simulink model "MPC_MG_raw_ver1"  (R2021b)
settings: Solver=ode23tb  StartTime=0.0  StopTime=1  RelTol=1e-3
model workspace (MAT data in the model file):
  Ts : Simulink.Parameter (value not decoded)
  secondary_on : Simulink.Parameter (value not decoded)
values from neighbouring files (symbols this model uses):
  A = zeros(4,4)    [MPC_MG_script_raw_dmpc.m]    (also in MPG_MG_July.m = [0 1 1 1; 1 0 0 0; 1 0 0 0; 1 0 0 0]; MPG_MG_freq_script.m = ones(4) - eye(4); Script.m = [0 1 1 1 ; 1 0 1 1 ; 1 1 0 1 ; 1 1 1 0])
  a12 = 0    [Four_DG_MG_PrimaryOnlyScript.m]    (also in MPC_MG_script_raw_dmpc.m; MPC_MG_secondary_script.m)
  a14 = 0    [Four_DG_MG_PrimaryOnlyScript.m]    (also in MPC_MG_script_raw_dmpc.m; MPC_MG_secondary_script.m)
  a21 = 1    [Four_DG_MG_PrimaryOnlyScript.m]    (also in MPC_MG_script_raw_dmpc.m; MPC_MG_secondary_script.m)
  a23 = 0    [Four_DG_MG_PrimaryOnlyScript.m]    (also in MPC_MG_script_raw_dmpc.m; MPC_MG_secondary_script.m)
  a32 = 1    [Four_DG_MG_PrimaryOnlyScript.m]    (also in MPC_MG_script_raw_dmpc.m; MPC_MG_secondary_script.m)
  a34 = 0    [Four_DG_MG_PrimaryOnlyScript.m]    (also in MPC_MG_script_raw_dmpc.m; MPC_MG_secondary_script.m)
  a41 = 1    [Four_DG_MG_PrimaryOnlyScript.m]    (also in MPC_MG_script_raw_dmpc.m; MPC_MG_secondary_script.m)
  a43 = 0    [Four_DG_MG_PrimaryOnlyScript.m]    (also in MPC_MG_script_raw_dmpc.m; MPC_MG_secondary_script.m)
  b1v = 1    [Four_DG_MG_PrimaryOnlyScript.m]    (also in MPC_MG_script_raw_dmpc.m; MPC_MG_secondary_script.m; MPG_MG_July.m; MPG_MG_freq_script.m)
  b1w = 1    [Four_DG_MG_PrimaryOnlyScript.m]    (also in MPC_MG_script_raw_dmpc.m; MPC_MG_secondary_script.m; MPG_MG_July.m; MPG_MG_freq_script.m)
  b2v = 0    [Four_DG_MG_PrimaryOnlyScript.m]    (also in MPC_MG_script_raw_dmpc.m; MPC_MG_secondary_script.m; MPG_MG_July.m; MPG_MG_freq_script.m)
  b2w = 0    [Four_DG_MG_PrimaryOnlyScript.m]    (also in MPC_MG_script_raw_dmpc.m; MPC_MG_secondary_script.m; MPG_MG_July.m; MPG_MG_freq_script.m)
  b3v = 0    [Four_DG_MG_PrimaryOnlyScript.m]    (also in MPC_MG_script_raw_dmpc.m; MPC_MG_secondary_script.m; MPG_MG_July.m; MPG_MG_freq_script.m)
  b3w = 0    [Four_DG_MG_PrimaryOnlyScript.m]    (also in MPC_MG_script_raw_dmpc.m; MPC_MG_secondary_script.m; MPG_MG_July.m; MPG_MG_freq_script.m)
  b4v = 0    [Four_DG_MG_PrimaryOnlyScript.m]    (also in MPC_MG_script_raw_dmpc.m; MPC_MG_secondary_script.m; MPG_MG_July.m; MPG_MG_freq_script.m)
  b4w = 0    [Four_DG_MG_PrimaryOnlyScript.m]    (also in MPC_MG_script_raw_dmpc.m; MPC_MG_secondary_script.m; MPG_MG_July.m; MPG_MG_freq_script.m)
  C_f = 50e-6    (= 5e-05)    [Four_DG_MG_PrimaryOnlyScript.m]    (also in MPC_MG_script.m; MPC_MG_script_raw_dmpc.m; MPC_MG_secondary_script.m; MPG_MG_July.m)
  cf = 60    [Four_DG_MG_PrimaryOnlyScript.m]    (also in MPC_MG_script_raw_dmpc.m = 40; MPC_MG_secondary_script.m = 40; MPG_MG_July.m = 100; MPG_MG_freq_script.m = 100)
  cv = 60    [Four_DG_MG_PrimaryOnlyScript.m]    (also in MPC_MG_script_raw_dmpc.m = 40; MPC_MG_secondary_script.m = 40; MPG_MG_July.m = 100; MPG_MG_freq_script.m = 100)
  f_c = 5000    [Four_DG_MG_PrimaryOnlyScript.m]    (also in MPC_MG_script.m = 40000; MPC_MG_script_raw_dmpc.m = 40000; MPC_MG_secondary_script.m = 40000; MPG_MG_July.m = 50000)
  kL = 1e-5    (= 1e-05)    [Four_DG_MG_PrimaryOnlyScript.m]    (also in MPC_MG_script.m = 1e-08; MPC_MG_script_raw_dmpc.m = 1e-08; MPC_MG_secondary_script.m = 1e-07; MPG_MG_July.m = 1e-07)
  L_f = 1.35e-3    (= 0.00135)    [Four_DG_MG_PrimaryOnlyScript.m]    (also in MPC_MG_script.m; MPC_MG_script_raw_dmpc.m; MPC_MG_secondary_script.m; MPG_MG_July.m)
  L_in1 = 0.35e-3    (= 0.00035)    [Four_DG_MG_PrimaryOnlyScript.m]    (also in MPC_MG_script.m; MPC_MG_script_raw_dmpc.m; MPC_MG_secondary_script.m; MPG_MG_July.m)
  L_in2 = 0.35e-3    (= 0.00035)    [Four_DG_MG_PrimaryOnlyScript.m]    (also in MPC_MG_script.m; MPC_MG_script_raw_dmpc.m; MPC_MG_secondary_script.m; MPG_MG_July.m)
  L_in3 = 0.35e-3    (= 0.00035)    [Four_DG_MG_PrimaryOnlyScript.m]    (also in MPC_MG_script.m; MPC_MG_script_raw_dmpc.m; MPC_MG_secondary_script.m; MPG_MG_July.m)
  lambda1 = [30000 50000 90000 50000]'    [MPC_MG_script_raw_dmpc.m]    (also in MPG_MG_July.m = [4 4 4 4]'; MPG_MG_freq_script.m = [3 3 3 3]'; Script.m = [1 1 1 1]')
  lambda2 = [5 6 7 6]'    [MPC_MG_script_raw_dmpc.m]    (also in MPG_MG_July.m = [0.5e-2 0.5e-2 0.5e-2 0.5e-2]'; MPG_MG_freq_script.m = [1.1 1.9 1.5 1.2]'; Script.m = [0.8e-2 0.8e-2 0.8e-2 0.8e-2]')
  lambda3 = [80000 80000 900000 80000]'    [MPC_MG_script_raw_dmpc.m]    (also in MPG_MG_July.m = [1e-3 1e-3 1e-3 1e-3]'; MPG_MG_freq_script.m = [9e-4 1.2e-2 3e-3 3e-3]'; Script.m = [1.5e-3 1.5e-3 1.5e-3 1.5e-3]')
  lambda4 = [5000 5000 5000 5000]'    [MPC_MG_script_raw_dmpc.m]
  lambda5 = [150 130 200 130]'    [MPC_MG_script_raw_dmpc.m]
  lambda6 = [5000 2000 1000 2000]'    [MPC_MG_script_raw_dmpc.m]
  LD_ref1 = 800e-6    (= 0.0008)    [Four_DG_MG_PrimaryOnlyScript.m]    (also in MPC_MG_script.m = 0.0003; MPC_MG_script_raw_dmpc.m = 0.0003; MPC_MG_secondary_script.m = 0.0001; MPG_MG_July.m = 0.0004)
  lo_co = 0.2    [Four_DG_MG_PrimaryOnlyScript.m]    (also in MPC_MG_script.m = 0.05; MPC_MG_script_raw_dmpc.m = 0.1; MPC_MG_secondary_script.m = 0.08; MPG_MG_July.m = 0.15)
  m_p1 = 9.4e-5/droopDivide    (= 9.4e-05)    [Four_DG_MG_PrimaryOnlyScript.m]    (also in MPC_MG_script.m; MPC_MG_script_raw_dmpc.m; MPC_MG_secondary_script.m; MPG_MG_July.m)
  m_p2 = 9.4e-5/droopDivide    (= 9.4e-05)    [Four_DG_MG_PrimaryOnlyScript.m]    (also in MPC_MG_script.m; MPC_MG_script_raw_dmpc.m; MPC_MG_secondary_script.m; MPG_MG_July.m)
  m_p3 = 12.5e-5/droopDivide    (= 0.000125)    [Four_DG_MG_PrimaryOnlyScript.m]    (also in MPC_MG_script.m; MPC_MG_script_raw_dmpc.m; MPC_MG_secondary_script.m; MPG_MG_July.m)
  m_p4 = 12.5e-5/droopDivide    (= 0.000125)    [Four_DG_MG_PrimaryOnlyScript.m]    (also in MPC_MG_script.m; MPC_MG_script_raw_dmpc.m; MPC_MG_secondary_script.m; MPG_MG_July.m)
  n_q1 = 1.3e-3/droopDivide2    (= 0.00013)    [Four_DG_MG_PrimaryOnlyScript.m]    (also in MPC_MG_script.m; MPC_MG_script_raw_dmpc.m; MPC_MG_secondary_script.m; MPG_MG_July.m)
  n_q2 = 1.3e-3/droopDivide2    (= 0.00013)    [Four_DG_MG_PrimaryOnlyScript.m]    (also in MPC_MG_script.m; MPC_MG_script_raw_dmpc.m; MPC_MG_secondary_script.m; MPG_MG_July.m)
  n_q3 = 1.5e-3/droopDivide2    (= 0.00015)    [Four_DG_MG_PrimaryOnlyScript.m]    (also in MPC_MG_script.m; MPC_MG_script_raw_dmpc.m; MPC_MG_secondary_script.m; MPG_MG_July.m)
  n_q4 = 1.5e-3/droopDivide2    (= 0.00015)    [Four_DG_MG_PrimaryOnlyScript.m]    (also in MPC_MG_script.m; MPC_MG_script_raw_dmpc.m; MPC_MG_secondary_script.m; MPG_MG_July.m)
  R_f = 0.1    [Four_DG_MG_PrimaryOnlyScript.m]    (also in MPC_MG_script.m; MPC_MG_script_raw_dmpc.m; MPC_MG_secondary_script.m; MPG_MG_July.m)
  R_in1 = 0.03    [Four_DG_MG_PrimaryOnlyScript.m]    (also in MPC_MG_script.m; MPC_MG_script_raw_dmpc.m; MPC_MG_secondary_script.m; MPG_MG_July.m)
  R_in2 = 0.03    [Four_DG_MG_PrimaryOnlyScript.m]    (also in MPC_MG_script.m; MPC_MG_script_raw_dmpc.m; MPC_MG_secondary_script.m; MPG_MG_July.m)
  R_in3 = 0.03    [Four_DG_MG_PrimaryOnlyScript.m]    (also in MPC_MG_script.m; MPC_MG_script_raw_dmpc.m; MPC_MG_secondary_script.m; MPG_MG_July.m)
  Smax = [45e3 45e3 37e3 37e3]'    [MPC_MG_script_raw_dmpc.m]
  Smax1 = 2400    [MPC_MG_script_raw_dmpc.m]
  Smax2 = 2400    [MPC_MG_script_raw_dmpc.m]
  Smax3 = 2400    [MPC_MG_script_raw_dmpc.m]
  Smax4 = 2400    [MPC_MG_script_raw_dmpc.m]
  time_thresh = 0.6    [Four_DG_MG_PrimaryOnlyScript.m]    (also in MPC_MG_script_raw_dmpc.m = 2; MPC_MG_secondary_script.m = 2; MPG_MG_July.m = 0.5; MPG_MG_freq_script.m = 0.5)
  Ts = 10e-6    (= 1e-05)    [Four_DG_MG_PrimaryOnlyScript.m]    (also in MPC_MG_script.m; MPC_MG_script_raw_dmpc.m; MPC_MG_secondary_script.m; MPG_MG_July.m)
  V_nom = 220*sqrt(2)    [Four_DG_MG_PrimaryOnlyScript.m]    (also in MPC_MG_script.m; MPC_MG_script_raw_dmpc.m; MPC_MG_secondary_script.m; MPG_MG_July.m)
  Vdc = 600    [Four_DG_MG_PrimaryOnlyScript.m]    (also in MPC_MG_script.m; MPC_MG_script_raw_dmpc.m; MPC_MG_secondary_script.m; MPG_MG_July.m)
  Vmax = 155    [MPC_MG_script_raw_dmpc.m]
  Vmin = 145    [MPC_MG_script_raw_dmpc.m]
  w_c_high = 2*pi*50    (= 314.159265359)    [Four_DG_MG_PrimaryOnlyScript.m]    (also in MPC_MG_script.m; MPC_MG_script_raw_dmpc.m; MPC_MG_secondary_script.m; MPG_MG_July.m)
  w_nom = 2*pi*50    (= 314.159265359)    [Four_DG_MG_PrimaryOnlyScript.m]    (also in MPC_MG_script.m; MPC_MG_script_raw_dmpc.m; MPC_MG_secondary_script.m; MPG_MG_July.m)
undefined symbols (not defined in the file or in its folder): i
libraries: spsThreePhaseSeriesRLCBranchLib x18, spsThreePhaseVIMeasurementLib x16, spsabctodq0Lib x16, eeGeneralControl x10, spsPLL3phLib x8, dspswit3 x5, powerlib x5, spsPMUPLLBasedPositiveSequenceLib x4, spsDCVoltageSourceLib x4, spsSeriesRLCBranchLib x4, spsTwoLevelConverterLib x4, spsThreePhaseSeriesRLCLoadLib x3
(part 4 of 4)

== matlab function MPC_MG_raw_ver1/Voltage Source Inverter 2/Model Predictive Control  ==
  settings: updateMethod=DISCRETE  sampleTime=Ts
  data: S_opt output; Sopt output size=[1 6]; Vc input; i_filter input; vref input; Vi_opt output; Vdc parameter double size=1; modT parameter size=1; Cfilter parameter size=1; Lfilter parameter size=1
function [S_opt, Sopt, Vi_opt] = MPC(Vc, i_filter,vref,Vdc,modT,Cfilter,Lfilter)

    % In order to call "cont2dis" function
    coder.extrinsic('cont2dis');
    persistent Aq Bq Bdq Vck ifk  Vc_old if_old x_opt g f_window f_window2

    % Initialize variables and get the parameters of the Discrete model based on Ts
    if isempty(x_opt), x_opt = ones(1, 2); end
    if isempty(Vc_old), Vc_old = 0 + 1j*0; end
    if isempty(if_old), if_old = 0 + 1j*0; end
    if isempty(Vck), Vck = ones(1, 4) * (0 + 1j*0); end
    if isempty(ifk), ifk = ones(1, 4) * (0 + 1j*0); end
    if isempty(f_window), f_window = zeros(1,51); end
    if isempty(f_window2), f_window2 = zeros(1,51); end

    if isempty(Aq) && isempty(Bq) && isempty(Bdq)
        Aq = zeros(2);     Bq = zeros(2,1);     Bdq = zeros(2,1);
        % Call "cont2dis" function
        [Aq, Bq, Bdq] = cont2dis(modT,Lfilter,Cfilter); 
    end
    
    % Intialize the cost function
    g_opt = inf;
    
    % To generate the switching states matrix
    states = [1 0 0;
              0 0 0  
              1 1 0
              0 1 0
              0 1 1
              0 0 1
              1 0 1
              1 1 1];
    a = exp(1j*(2*pi/3));
    % Read current measurements at sampling instant k
    ifk(1) = i_filter;
    Vck(1) = Vc;
    % Equation of io(k-1) = if(k-1)-(c/Ts)(vc(k)-vc(k-1)).
    io = ones(1, 3) * (0 + 1j*0);
    io(1) = if_old - (Cfilter/modT)*(Vck(1) - Vc_old); 
    
    % Store the measured current for the next iteration
    if_old = i_filter;
    Vc_old = Vc;
    % FOR loop to find the best switch in the next instant and its corresponding V(i)
    k = ones(1,3);
    s = zeros(3,3);
    sw = zeros(1,3)* (0 + 1j*0);
    Vi = zeros(1,3)* (0 + 1j*0);
    for a1 = 1:8
        k(1) = a1;
        %constraint check
        if (abs(states(k(1),:)-states(x_opt(1),:)) > 1)
            continue
        end
        %state calculation
        s(1,:) = states(k(1),:);
        sw(1) = (2/3)*(s(1,1)+a*s(1,2)+a^2*s(1,3));
        Vi(1) = Vdc*sw(1);

        % Output Voltage Prediction at instant k+1
        ifk(2) = Aq(1,1)*ifk(1) + Aq(1,2)*Vck(1) + Bq(1)*Vi(1) + Bdq(1)*io(1); 
        Vck(2) = Aq(2,1)*ifk(1) + Aq(2,2)*Vck(1) + Bq(2)*Vi(1) + Bdq(2)*io(1); 
        
        for a2 = 1:8
            k(2) = a2;
            %constraint check
            if (abs(states(k(2),:)-states(k(1),:)) > 1)
                continue
            end
            io(2) = io(1) - (Cfilter/modT)*(Vck(2) - Vck(1));
            %state calculation
            s(2,:) = states(k(2),:);
            sw(2) = (2/3)*(s(2,1)+a*s(2,2)+a^2*s(2,3));
            Vi(2) = Vdc*sw(2);
    
            % Output Voltage Prediction at instant k+1
            ifk(3) = Aq(1,1)*ifk(2) + Aq(1,2)*Vck(2) + Bq(1)*Vi(2) + Bdq(1)*io(2); 
            Vck(3) = Aq(2,1)*ifk(2) + Aq(2,2)*Vck(2) + Bq(2)*Vi(2) + Bdq(2)*io(2); 

            g1 = (real(ifk(3))-real(io(3))+Cfilter*2*pi*50*imag(vref))^2 + (imag(ifk(3))-imag(io(3))+Cfilter*2*pi*50*real(vref))^2;
            g = (real(vref)-real(Vck(3)))^2+(imag(vref)-imag(Vck(3)))^2 + 0.1*g1;
            if (g<g_opt)
                x_opt = [k(1) k(2)];
                g_opt = g;
            end
           
        end 
    end

     
    
    % Output switching states and its voltage vector. 
    Vi_opt = x_opt(1); 
    S_opt = states(x_opt(1),:);
    d_opt = not(S_opt);
    Sopt = [S_opt,d_opt];     

end

== matlab function MPC_MG_raw_ver1/Voltage Source Inverter 1/Model Predictive Control  ==
  settings: updateMethod=DISCRETE  sampleTime=Ts
  data: S_opt output; Sopt output size=[1 6]; Vc input; i_filter input; vref input; Vi_opt output; Vdc parameter double size=1; modT parameter size=1; Cfilter parameter size=1; Lfilter parameter size=1
function [S_opt, Sopt, Vi_opt] = MPC(Vc, i_filter,vref,Vdc,modT,Cfilter,Lfilter)

    % In order to call "cont2dis" function
    coder.extrinsic('cont2dis');
    persistent Aq Bq Bdq Vck ifk  Vc_old if_old x_opt g f_window f_window2

    % Initialize variables and get the parameters of the Discrete model based on Ts
    if isempty(x_opt), x_opt = ones(1, 2); end
    if isempty(Vc_old), Vc_old = 0 + 1j*0; end
    if isempty(if_old), if_old = 0 + 1j*0; end
    if isempty(Vck), Vck = ones(1, 4) * (0 + 1j*0); end
    if isempty(ifk), ifk = ones(1, 4) * (0 + 1j*0); end
    if isempty(f_window), f_window = zeros(1,51); end
    if isempty(f_window2), f_window2 = zeros(1,51); end

    if isempty(Aq) && isempty(Bq) && isempty(Bdq)
        Aq = zeros(2);     Bq = zeros(2,1);     Bdq = zeros(2,1);
        % Call "cont2dis" function
        [Aq, Bq, Bdq] = cont2dis(modT,Lfilter,Cfilter); 
    end
    
    % Intialize the cost function
    g_opt = inf;
    
    % To generate the switching states matrix
    states = [1 0 0;
              0 0 0  
              1 1 0
              0 1 0
              0 1 1
              0 0 1
              1 0 1
              1 1 1];
    a = exp(1j*(2*pi/3));
    % Read current measurements at sampling instant k
    ifk(1) = i_filter;
    Vck(1) = Vc;
    % Equation of io(k-1) = if(k-1)-(c/Ts)(vc(k)-vc(k-1)).
    io = ones(1, 3) * (0 + 1j*0);
    io(1) = if_old - (Cfilter/modT)*(Vck(1) - Vc_old); 
    
    % Store the measured current for the next iteration
    if_old = i_filter;
    Vc_old = Vc;
    % FOR loop to find the best switch in the next instant and its corresponding V(i)
    k = ones(1,3);
    s = zeros(3,3);
    sw = zeros(1,3)* (0 + 1j*0);
    Vi = zeros(1,3)* (0 + 1j*0);
    for a1 = 1:8
        k(1) = a1;
        %constraint check
        if (abs(states(k(1),:)-states(x_opt(1),:)) > 1)
            continue
        end
        %state calculation
        s(1,:) = states(k(1),:);
        sw(1) = (2/3)*(s(1,1)+a*s(1,2)+a^2*s(1,3));
        Vi(1) = Vdc*sw(1);

        % Output Voltage Prediction at instant k+1
        ifk(2) = Aq(1,1)*ifk(1) + Aq(1,2)*Vck(1) + Bq(1)*Vi(1) + Bdq(1)*io(1); 
        Vck(2) = Aq(2,1)*ifk(1) + Aq(2,2)*Vck(1) + Bq(2)*Vi(1) + Bdq(2)*io(1); 
        
        for a2 = 1:8
            k(2) = a2;
            %constraint check
            if (abs(states(k(2),:)-states(k(1),:)) > 1)
                continue
            end
            io(2) = io(1) - (Cfilter/modT)*(Vck(2) - Vck(1));
            %state calculation
            s(2,:) = states(k(2),:);
            sw(2) = (2/3)*(s(2,1)+a*s(2,2)+a^2*s(2,3));
            Vi(2) = Vdc*sw(2);
    
            % Output Voltage Prediction at instant k+1
            ifk(3) = Aq(1,1)*ifk(2) + Aq(1,2)*Vck(2) + Bq(1)*Vi(2) + Bdq(1)*io(2); 
            Vck(3) = Aq(2,1)*ifk(2) + Aq(2,2)*Vck(2) + Bq(2)*Vi(2) + Bdq(2)*io(2); 

            g1 = (real(ifk(3))-real(io(3))+Cfilter*2*pi*50*imag(vref))^2 + (imag(ifk(3))-imag(io(3))+Cfilter*2*pi*50*real(vref))^2;
            g = (real(vref)-real(Vck(3)))^2+(imag(vref)-imag(Vck(3)))^2 + 0.1*g1;
            if (g<g_opt)
                x_opt = [k(1) k(2)];
                g_opt = g;
            end
           
        end 
    end

     
    
    % Output switching states and its voltage vector. 
    Vi_opt = x_opt(1); 
    S_opt = states(x_opt(1),:);
    d_opt = not(S_opt);
    Sopt = [S_opt,d_opt];     

end

== matlab function MPC_MG_raw_ver1/Voltage Source Inverter 3/Model Predictive Control  ==
  settings: updateMethod=DISCRETE  sampleTime=Ts
  data: S_opt output; Sopt output size=[1 6]; Vc input; i_filter input; vref input; Vi_opt output; Vdc parameter double size=1; modT parameter size=1; Cfilter parameter size=1; Lfilter parameter size=1
function [S_opt, Sopt, Vi_opt] = MPC(Vc, i_filter,vref,Vdc,modT,Cfilter,Lfilter)

    % In order to call "cont2dis" function
    coder.extrinsic('cont2dis');
    persistent Aq Bq Bdq Vck ifk  Vc_old if_old x_opt g f_window f_window2

    % Initialize variables and get the parameters of the Discrete model based on Ts
    if isempty(x_opt), x_opt = ones(1, 2); end
    if isempty(Vc_old), Vc_old = 0 + 1j*0; end
    if isempty(if_old), if_old = 0 + 1j*0; end
    if isempty(Vck), Vck = ones(1, 4) * (0 + 1j*0); end
    if isempty(ifk), ifk = ones(1, 4) * (0 + 1j*0); end
    if isempty(f_window), f_window = zeros(1,51); end
    if isempty(f_window2), f_window2 = zeros(1,51); end

    if isempty(Aq) && isempty(Bq) && isempty(Bdq)
        Aq = zeros(2);     Bq = zeros(2,1);     Bdq = zeros(2,1);
        % Call "cont2dis" function
        [Aq, Bq, Bdq] = cont2dis(modT,Lfilter,Cfilter); 
    end
    
    % Intialize the cost function
    g_opt = inf;
    
    % To generate the switching states matrix
    states = [1 0 0;
              0 0 0  
              1 1 0
              0 1 0
              0 1 1
              0 0 1
              1 0 1
              1 1 1];
    a = exp(1j*(2*pi/3));
    % Read current measurements at sampling instant k
    ifk(1) = i_filter;
    Vck(1) = Vc;
    % Equation of io(k-1) = if(k-1)-(c/Ts)(vc(k)-vc(k-1)).
    io = ones(1, 3) * (0 + 1j*0);
    io(1) = if_old - (Cfilter/modT)*(Vck(1) - Vc_old); 
    
    % Store the measured current for the next iteration
    if_old = i_filter;
    Vc_old = Vc;
    % FOR loop to find the best switch in the next instant and its corresponding V(i)
    k = ones(1,3);
    s = zeros(3,3);
    sw = zeros(1,3)* (0 + 1j*0);
    Vi = zeros(1,3)* (0 + 1j*0);
    for a1 = 1:8
        k(1) = a1;
        %constraint check
        if (abs(states(k(1),:)-states(x_opt(1),:)) > 1)
            continue
        end
        %state calculation
        s(1,:) = states(k(1),:);
        sw(1) = (2/3)*(s(1,1)+a*s(1,2)+a^2*s(1,3));
        Vi(1) = Vdc*sw(1);

        % Output Voltage Prediction at instant k+1
        ifk(2) = Aq(1,1)*ifk(1) + Aq(1,2)*Vck(1) + Bq(1)*Vi(1) + Bdq(1)*io(1); 
        Vck(2) = Aq(2,1)*ifk(1) + Aq(2,2)*Vck(1) + Bq(2)*Vi(1) + Bdq(2)*io(1); 
        
        for a2 = 1:8
            k(2) = a2;
            %constraint check
            if (abs(states(k(2),:)-states(k(1),:)) > 1)
                continue
            end
            io(2) = io(1) - (Cfilter/modT)*(Vck(2) - Vck(1));
            %state calculation
            s(2,:) = states(k(2),:);
            sw(2) = (2/3)*(s(2,1)+a*s(2,2)+a^2*s(2,3));
            Vi(2) = Vdc*sw(2);
    
            % Output Voltage Prediction at instant k+1
            ifk(3) = Aq(1,1)*ifk(2) + Aq(1,2)*Vck(2) + Bq(1)*Vi(2) + Bdq(1)*io(2); 
            Vck(3) = Aq(2,1)*ifk(2) + Aq(2,2)*Vck(2) + Bq(2)*Vi(2) + Bdq(2)*io(2); 

            g1 = (real(ifk(3))-real(io(3))+Cfilter*2*pi*50*imag(vref))^2 + (imag(ifk(3))-imag(io(3))+Cfilter*2*pi*50*real(vref))^2;
            g = (real(vref)-real(Vck(3)))^2+(imag(vref)-imag(Vck(3)))^2 + 0.1*g1;
            if (g<g_opt)
                x_opt = [k(1) k(2)];
                g_opt = g;
            end
           
        end 
    end

     
    
    % Output switching states and its voltage vector. 
    Vi_opt = x_opt(1); 
    S_opt = states(x_opt(1),:);
    d_opt = not(S_opt);
    Sopt = [S_opt,d_opt];     

end

== matlab function MPC_MG_raw_ver1/MPC-based Secondary Controller/Model Predictive Control 1 ==
  settings: updateMethod=DISCRETE  sampleTime=Ts
  data: L_f input; Mpw input; Mqv input; Tsec input; omega input; omega_s input; V input; V_s input; theta input; d_omega output; d_V output size=[1 6]; P input; Q input; a input; Vmin input; Vmax input; w_nom input; V_nom input; lambda1 input; lambda2 input; lambda3 input; lambda4 input; lambda5 input; lambda6 input; Smax input; aij input
function [d_omega, d_V] = fcn(L_f, Mpw, Mqv, Tsec, omega, omega_s, V, V_s, theta, P, Q, a, Vmin, Vmax, w_nom, V_nom, lambda1, lambda2, lambda3, lambda4, lambda5, lambda6, Smax, aij)
    persistent omega_k V_k theta_k P_k Q_k d_omega_old d_V_old;
    
    if isempty(omega_k), omega_k = 0; end
    if isempty(V_k), V_k = 0; end
    if isempty(theta_k), theta_k = 0; end
    if isempty(P_k), P_k = 0; end
    if isempty(Q_k), Q_k = 0; end
    if isempty(d_omega_old), d_omega_old = 0; end
    if isempty(d_V_old), d_V_old = 0; end
    %all inputs are 4-element vector
    %step 4:
    %omega_overline = (omega(a) + aij(a,:)*omega)/ (1+aij(a,:));
    %V_overline = (V(a) + aij(a,:)*V)/ (1+aij(a,:));
    %step 5: update matrices
    Ai = zeros(3,9);
    Ai(1,4) = 1;
    Ai(2,4) = -1;
    Ai(3,5) = sign(P(a));
    Ai(3,6) = sign(Q(a));
    
    Bi = zeros(3,1);
    Bi(1,1) = Vmin;
    Bi(2,1) = -Vmax;
    Bi(3,1) = Smax(a) -(abs(P(a))+abs(Q(a))) + sign(P(a))*P(a) + sign(Q(a))*Q(a);

    omega_k = omega(a) + Mpw*(P_k - P(a)) + d_omega_old;
    V_k = V(a) + Mqv*(Q_k - Q(a)) + d_V_old;
    theta_k = theta + Tsec*(omega_k - omega_s(a));
    P_k = P(a) + (V_k - V(a))/(L_f*w_nom)*V_s(a)*sin(theta(a)) + (theta_k-theta(a))/(L_f*w_nom)*V(a)*V_s(a)*cos(theta(a));
    Q_k = Q(a) + (V_k - V(a))/(L_f*w_nom)*(2*V(a)-V_s(a)*cos(theta(a))) + (theta_k-theta(a))/(L_f*w_nom)*V(a)*V_s(a)*sin(theta(a));
    Aeq = eye(7,9);
    Beq = [w_nom; V_nom; omega_k; V_k; theta_k; P_k; Q_k ; 0; 0];
    
    H = zeros(9);
    H(1,1) = 2*lambda1(a);
    H(2,2) = 2*lambda2(a);
    H(6,6) = 2*lambda5(a)/Smax(a);
    H(7,7) = H(6,6)*lambda6(a)/lambda5(a);
    H(8,8) = 2*lambda3(a);
    H(9,9) = 2*lambda4(a);
    
    F = zeros(9,1);
    F(1,1) = -2*lambda1(a);
    F(2,1) = -2*lambda2(a);
    F(6,1) = -2*lambda5(a)*sum(aij(a,:)*P/Smax)*P(a)/Smax(a);
    F(7,1) = -2*lambda6(a)*sum(aij(a,:)*P/Smax)*P(a)/Smax(a);

    options = optimoptions('quadprog','Display','iter');

    [x, exitflag] = quadprog(H, F, Ai, Bi, Aeq, Beq, [], [], [], options);

    if exitflag > 0
        d_omega = x(8);
        d_V = x(9);
    else
        d_omega = 0;
        d_V = 0;
    end
    d_omega_old = d_omega;
    d_V_old = d_V;
    
end

== matlab function MPC_MG_raw_ver1/Voltage Source Inverter 5/Model Predictive Control  ==
  settings: updateMethod=DISCRETE  sampleTime=Ts
  data: S_opt output; Sopt output size=[1 6]; Vc input; i_filter input; vref input; Vi_opt output; Vdc parameter double size=1; modT parameter size=1; Cfilter parameter size=1; Lfilter parameter size=1
function [S_opt, Sopt, Vi_opt] = MPC(Vc, i_filter,vref,Vdc,modT,Cfilter,Lfilter)

    % In order to call "cont2dis" function
    coder.extrinsic('cont2dis');
    persistent Aq Bq Bdq Vc1 if1 Vc_old if_old x_opt g f_window f_window2 fil fil2

    % Initialize variables and get the parameters of the Discrete model based on Ts
    if isempty(x_opt), x_opt = 1; end
    if isempty(Vc1), Vc1 = 0 + 1j*0; end
    if isempty(Vc_old), Vc_old = 0 + 1j*0; end
    if isempty(if_old), if_old = 0 + 1j*0; end
    if isempty(if1), if1 = 0 + 1j*0; end
    if isempty(f_window), f_window = zeros(1,51); end
    if isempty(f_window2), f_window2 = zeros(1,51); end

    if isempty(Aq) && isempty(Bq) && isempty(Bdq)
        Aq = zeros(2);     Bq = zeros(2,1);     Bdq = zeros(2,1);
        % Call "cont2dis" function
        [Aq, Bq, Bdq] = cont2dis(modT,Lfilter,Cfilter); 
    end
    
    % Intialize the cost function
    g_opt = inf;
    
    % To generate the switching states matrix
    states = [1 0 0;
              0 0 0  
              1 1 0
              0 1 0
              0 1 1
              0 0 1
              1 0 1
              1 1 1];
    a = exp(1j*(2*pi/3));
    %notch filter
    fil = fir1(2,[0.1225 0.1275],'DC-0');
    fil2 = fir1(2,[0.1225 0.1275],'DC-0');
    
    % Read current measurements at sampling instant k
    ifk = i_filter;
    Vck = Vc;
    % Equation of io(k-1) = if(k-1)-(c/Ts)(vc(k)-vc(k-1)).
    io = if_old - (Cfilter/modT)*(Vck - Vc_old); 
    
    % Store the measured current for the next iteration
    if_old = ifk;
    Vc_old = Vck;
    % FOR loop to find the best switch in the next instant and its corresponding V(i)
    for k = 1:8
        s = states(k,:);
        sw = (2/3)*(s(1)+a*s(2)+a^2*s(3));
        Vi = Vdc*sw;

        % Output Voltage Prediction at instant k+1
        if1 = Aq(1,1)*ifk + Aq(1,2)*Vck + Bq(1)*Vi + Bdq(1)*io; 
        Vc1 = Aq(2,1)*ifk + Aq(2,2)*Vck + Bq(2)*Vi + Bdq(2)*io; 
        Nc = sum(abs(states(k,:)-states(x_opt,:)))^2;    
        gf = filter(fil, 1, f_window);
        gf2 = filter(fil2, 1, f_window2);
        g1 = (real(if1)-real(io)+Cfilter*2*pi*50*imag(vref))^2 + (imag(if1)-imag(io)+Cfilter*2*pi*50*real(vref))^2;
        g = (real(vref)-real(Vc1))^2+(imag(vref)-imag(Vc1))^2 + 0.1*g1 + 3*Nc + 3*gf(1) + 3*gf2(1);
        if (g < g_opt)
            x_opt = k;
            g_opt = g;
            f_window = [sqrt((real(vref)-real(Vc1))^2+(imag(vref)-imag(Vc1))^2), f_window(1:(length(f_window)-1))];
            f_window2 = [g, f_window2(1:(length(f_window2)-1))];
        end
             
    end
    
    % Output switching states and its voltage vector. 
    Vi_opt = x_opt; 
    S_opt = states(x_opt,:);
    d_opt = not(S_opt);
    Sopt = [S_opt,d_opt];     

end

== matlab function MPC_MG_raw_ver1/MPC-based Secondary Controller/Model Predictive Control 2 ==
  settings: updateMethod=DISCRETE  sampleTime=Ts
  data: L_f input; Mpw input; Mqv input; Tsec input; omega input; omega_s input; V input; V_s input; theta input; d_omega output; d_V output size=[1 6]; P input; Q input; a input; Vmin input; Vmax input; w_nom input; V_nom input; lambda1 input; lambda2 input; lambda3 input; lambda4 input; lambda5 input; lambda6 input; Smax input; aij input
function [d_omega, d_V] = fcn(L_f, Mpw, Mqv, Tsec, omega, omega_s, V, V_s, theta, P, Q, a, Vmin, Vmax, w_nom, V_nom, lambda1, lambda2, lambda3, lambda4, lambda5, lambda6, Smax, aij)
    persistent omega_k V_k theta_k P_k Q_k d_omega_old d_V_old;
    
    if isempty(omega_k), omega_k = 0; end
    if isempty(V_k), V_k = 0; end
    if isempty(theta_k), theta_k = 0; end
    if isempty(P_k), P_k = 0; end
    if isempty(Q_k), Q_k = 0; end
    if isempty(d_omega_old), d_omega_old = 0; end
    if isempty(d_V_old), d_V_old = 0; end
    %all inputs are 4-element vector
    %step 4:
    %omega_overline = (omega(a) + aij(a,:)*omega)/ (1+aij(a,:));
    %V_overline = (V(a) + aij(a,:)*V)/ (1+aij(a,:));
    %step 5: update matrices
    Ai = zeros(3,9);
    Ai(1,4) = 1;
    Ai(2,4) = -1;
    Ai(3,5) = sign(P(a));
    Ai(3,6) = sign(Q(a));
    
    Bi = zeros(3,1);
    Bi(1,1) = Vmin;
    Bi(2,1) = -Vmax;
    Bi(3,1) = Smax(a) -(abs(P(a))+abs(Q(a))) + sign(P(a))*P(a) + sign(Q(a))*Q(a);

    omega_k = omega(a) + Mpw*(P_k - P(a)) + d_omega_old;
    V_k = V(a) + Mqv*(Q_k - Q(a)) + d_V_old;
    theta_k = theta + Tsec*(omega_k - omega_s(a));
    P_k = P(a) + (V_k - V(a))/(L_f*w_nom)*V_s(a)*sin(theta(a)) + (theta_k-theta(a))/(L_f*w_nom)*V(a)*V_s(a)*cos(theta(a));
    Q_k = Q(a) + (V_k - V(a))/(L_f*w_nom)*(2*V(a)-V_s(a)*cos(theta(a))) + (theta_k-theta(a))/(L_f*w_nom)*V(a)*V_s(a)*sin(theta(a));
    Aeq = eye(7,9);
    Beq = [w_nom; V_nom; omega_k; V_k; theta_k; P_k; Q_k ; 0; 0];
    
    H = zeros(9);
    H(1,1) = 2*lambda1(a);
    H(2,2) = 2*lambda2(a);
    H(6,6) = 2*lambda5(a)/Smax(a);
    H(7,7) = H(6,6)*lambda6(a)/lambda5(a);
    H(8,8) = 2*lambda3(a);
    H(9,9) = 2*lambda4(a);
    
    F = zeros(9,1);
    F(1,1) = -2*lambda1(a);
    F(2,1) = -2*lambda2(a);
    F(6,1) = -2*lambda5(a)*sum(aij(a,:)*P/Smax)*P(a)/Smax(a);
    F(7,1) = -2*lambda6(a)*sum(aij(a,:)*P/Smax)*P(a)/Smax(a);

    options = optimoptions('quadprog','Display','iter');

    [x, exitflag] = quadprog(H, F, Ai, Bi, Aeq, Beq, [], [], [], options);

    if exitflag > 0
        d_omega = x(8);
        d_V = x(9);
    else
        d_omega = 0;
        d_V = 0;
    end
    d_omega_old = d_omega;
    d_V_old = d_V;
    
end

== matlab function MPC_MG_raw_ver1/MPC-based Secondary Controller/Model Predictive Control 3 ==
  settings: updateMethod=DISCRETE  sampleTime=Ts
  data: L_f input; Mpw input; Mqv input; Tsec input; omega input; omega_s input; V input; V_s input; theta input; d_omega output; d_V output size=[1 6]; P input; Q input; a input; Vmin input; Vmax input; w_nom input; V_nom input; lambda1 input; lambda2 input; lambda3 input; lambda4 input; lambda5 input; lambda6 input; Smax input; aij input
function [d_omega, d_V] = fcn(L_f, Mpw, Mqv, Tsec, omega, omega_s, V, V_s, theta, P, Q, a, Vmin, Vmax, w_nom, V_nom, lambda1, lambda2, lambda3, lambda4, lambda5, lambda6, Smax, aij)
    persistent omega_k V_k theta_k P_k Q_k d_omega_old d_V_old;
    
    if isempty(omega_k), omega_k = 0; end
    if isempty(V_k), V_k = 0; end
    if isempty(theta_k), theta_k = 0; end
    if isempty(P_k), P_k = 0; end
    if isempty(Q_k), Q_k = 0; end
    if isempty(d_omega_old), d_omega_old = 0; end
    if isempty(d_V_old), d_V_old = 0; end
    %all inputs are 4-element vector
    %step 4:
    %omega_overline = (omega(a) + aij(a,:)*omega)/ (1+aij(a,:));
    %V_overline = (V(a) + aij(a,:)*V)/ (1+aij(a,:));
    %step 5: update matrices
    Ai = zeros(3,9);
    Ai(1,4) = 1;
    Ai(2,4) = -1;
    Ai(3,5) = sign(P(a));
    Ai(3,6) = sign(Q(a));
    
    Bi = zeros(3,1);
    Bi(1,1) = Vmin;
    Bi(2,1) = -Vmax;
    Bi(3,1) = Smax(a) -(abs(P(a))+abs(Q(a))) + sign(P(a))*P(a) + sign(Q(a))*Q(a);

    omega_k = omega(a) + Mpw*(P_k - P(a)) + d_omega_old;
    V_k = V(a) + Mqv*(Q_k - Q(a)) + d_V_old;
    theta_k = theta + Tsec*(omega_k - omega_s(a));
    P_k = P(a) + (V_k - V(a))/(L_f*w_nom)*V_s(a)*sin(theta(a)) + (theta_k-theta(a))/(L_f*w_nom)*V(a)*V_s(a)*cos(theta(a));
    Q_k = Q(a) + (V_k - V(a))/(L_f*w_nom)*(2*V(a)-V_s(a)*cos(theta(a))) + (theta_k-theta(a))/(L_f*w_nom)*V(a)*V_s(a)*sin(theta(a));
    Aeq = eye(7,9);
    Beq = [w_nom; V_nom; omega_k; V_k; theta_k; P_k; Q_k ; 0; 0];
    
    H = zeros(9);
    H(1,1) = 2*lambda1(a);
    H(2,2) = 2*lambda2(a);
    H(6,6) = 2*lambda5(a)/Smax(a);
    H(7,7) = H(6,6)*lambda6(a)/lambda5(a);
    H(8,8) = 2*lambda3(a);
    H(9,9) = 2*lambda4(a);
    
    F = zeros(9,1);
    F(1,1) = -2*lambda1(a);
    F(2,1) = -2*lambda2(a);
    F(6,1) = -2*lambda5(a)*sum(aij(a,:)*P/Smax)*P(a)/Smax(a);
    F(7,1) = -2*lambda6(a)*sum(aij(a,:)*P/Smax)*P(a)/Smax(a);

    options = optimoptions('quadprog','Display','iter');

    [x, exitflag] = quadprog(H, F, Ai, Bi, Aeq, Beq, [], [], [], options);

    if exitflag > 0
        d_omega = x(8);
        d_V = x(9);
    else
        d_omega = 0;
        d_V = 0;
    end
    d_omega_old = d_omega;
    d_V_old = d_V;
    
end

== matlab function MPC_MG_raw_ver1/Voltage Source Inverter 4/Model Predictive Control  ==
  settings: updateMethod=DISCRETE  sampleTime=Ts
  data: S_opt output; Sopt output size=[1 6]; Vc input; i_filter input; vref input; Vi_opt output; Vdc parameter double size=1; modT parameter size=1; Cfilter parameter size=1; Lfilter parameter size=1
function [S_opt, Sopt, Vi_opt] = MPC(Vc, i_filter,vref,Vdc,modT,Cfilter,Lfilter)

    % In order to call "cont2dis" function
    coder.extrinsic('cont2dis');
    persistent Aq Bq Bdq Vck ifk  Vc_old if_old x_opt g f_window f_window2

    % Initialize variables and get the parameters of the Discrete model based on Ts
    if isempty(x_opt), x_opt = ones(1, 2); end
    if isempty(Vc_old), Vc_old = 0 + 1j*0; end
    if isempty(if_old), if_old = 0 + 1j*0; end
    if isempty(Vck), Vck = ones(1, 4) * (0 + 1j*0); end
    if isempty(ifk), ifk = ones(1, 4) * (0 + 1j*0); end
    if isempty(f_window), f_window = zeros(1,51); end
    if isempty(f_window2), f_window2 = zeros(1,51); end

    if isempty(Aq) && isempty(Bq) && isempty(Bdq)
        Aq = zeros(2);     Bq = zeros(2,1);     Bdq = zeros(2,1);
        % Call "cont2dis" function
        [Aq, Bq, Bdq] = cont2dis(modT,Lfilter,Cfilter); 
    end
    
    % Intialize the cost function
    g_opt = inf;
    
    % To generate the switching states matrix
    states = [1 0 0;
              0 0 0  
              1 1 0
              0 1 0
              0 1 1
              0 0 1
              1 0 1
              1 1 1];
    a = exp(1j*(2*pi/3));
    % Read current measurements at sampling instant k
    ifk(1) = i_filter;
    Vck(1) = Vc;
    % Equation of io(k-1) = if(k-1)-(c/Ts)(vc(k)-vc(k-1)).
    io = ones(1, 3) * (0 + 1j*0);
    io(1) = if_old - (Cfilter/modT)*(Vck(1) - Vc_old); 
    
    % Store the measured current for the next iteration
    if_old = i_filter;
    Vc_old = Vc;
    % FOR loop to find the best switch in the next instant and its corresponding V(i)
    k = ones(1,3);
    s = zeros(3,3);
    sw = zeros(1,3)* (0 + 1j*0);
    Vi = zeros(1,3)* (0 + 1j*0);
    for a1 = 1:8
        k(1) = a1;
        %constraint check
        if (abs(states(k(1),:)-states(x_opt(1),:)) > 1)
            continue
        end
        %state calculation
        s(1,:) = states(k(1),:);
        sw(1) = (2/3)*(s(1,1)+a*s(1,2)+a^2*s(1,3));
        Vi(1) = Vdc*sw(1);

        % Output Voltage Prediction at instant k+1
        ifk(2) = Aq(1,1)*ifk(1) + Aq(1,2)*Vck(1) + Bq(1)*Vi(1) + Bdq(1)*io(1); 
        Vck(2) = Aq(2,1)*ifk(1) + Aq(2,2)*Vck(1) + Bq(2)*Vi(1) + Bdq(2)*io(1); 
        
        for a2 = 1:8
            k(2) = a2;
            %constraint check
            if (abs(states(k(2),:)-states(k(1),:)) > 1)
                continue
            end
            io(2) = io(1) - (Cfilter/modT)*(Vck(2) - Vck(1));
            %state calculation
            s(2,:) = states(k(2),:);
            sw(2) = (2/3)*(s(2,1)+a*s(2,2)+a^2*s(2,3));
            Vi(2) = Vdc*sw(2);
    
            % Output Voltage Prediction at instant k+1
            ifk(3) = Aq(1,1)*ifk(2) + Aq(1,2)*Vck(2) + Bq(1)*Vi(2) + Bdq(1)*io(2); 
            Vck(3) = Aq(2,1)*ifk(2) + Aq(2,2)*Vck(2) + Bq(2)*Vi(2) + Bdq(2)*io(2); 

            g1 = (real(ifk(3))-real(io(3))+Cfilter*2*pi*50*imag(vref))^2 + (imag(ifk(3))-imag(io(3))+Cfilter*2*pi*50*real(vref))^2;
            g = (real(vref)-real(Vck(3)))^2+(imag(vref)-imag(Vck(3)))^2 + 0.1*g1;
            if (g<g_opt)
                x_opt = [k(1) k(2)];
                g_opt = g;
            end
           
        end 
    end

     
    
    % Output switching states and its voltage vector. 
    Vi_opt = x_opt(1); 
    S_opt = states(x_opt(1),:);
    d_opt = not(S_opt);
    Sopt = [S_opt,d_opt];     

end

== matlab function MPC_MG_raw_ver1/MPC-based Secondary Controller/Model Predictive Control  ==
  settings: updateMethod=DISCRETE  sampleTime=Ts
  data: L_f input; Mpw input; Mqv input; Tsec input; omega input; omega_s input; V input; V_s input; theta input; d_omega output; d_V output size=[1 6]; P input; Q input; a input; Vmin input; Vmax input; w_nom input; V_nom input; lambda1 input; lambda2 input; lambda3 input; lambda4 input; lambda5 input; lambda6 input; Smax input; aij input
function [d_omega, d_V] = fcn(L_f, Mpw, Mqv, Tsec, omega, omega_s, V, V_s, theta, P, Q, a, Vmin, Vmax, w_nom, V_nom, lambda1, lambda2, lambda3, lambda4, lambda5, lambda6, Smax, aij)
    persistent omega_k V_k theta_k P_k Q_k d_omega_old d_V_old;
    
    if isempty(omega_k), omega_k = 0; end
    if isempty(V_k), V_k = 0; end
    if isempty(theta_k), theta_k = 0; end
    if isempty(P_k), P_k = 0; end
    if isempty(Q_k), Q_k = 0; end
    if isempty(d_omega_old), d_omega_old = 0; end
    if isempty(d_V_old), d_V_old = 0; end
    %all inputs are 4-element vector
    %step 4:
    %omega_overline = (omega(a) + aij(a,:)*omega)/ (1+aij(a,:));
    %V_overline = (V(a) + aij(a,:)*V)/ (1+aij(a,:));
    %step 5: update matrices
    Ai = zeros(3,9);
    Ai(1,4) = 1;
    Ai(2,4) = -1;
    Ai(3,5) = sign(P(a));
    Ai(3,6) = sign(Q(a));
    
    Bi = zeros(3,1);
    Bi(1,1) = Vmin;
    Bi(2,1) = -Vmax;
    Bi(3,1) = Smax(a) -(abs(P(a))+abs(Q(a))) + sign(P(a))*P(a) + sign(Q(a))*Q(a);

    omega_k = omega(a) + Mpw*(P_k - P(a)) + d_omega_old;
    V_k = V(a) + Mqv*(Q_k - Q(a)) + d_V_old;
    theta_k = theta + Tsec*(omega_k - omega_s(a));
    P_k = P(a) + (V_k - V(a))/(L_f*w_nom)*V_s(a)*sin(theta(a)) + (theta_k-theta(a))/(L_f*w_nom)*V(a)*V_s(a)*cos(theta(a));
    Q_k = Q(a) + (V_k - V(a))/(L_f*w_nom)*(2*V(a)-V_s(a)*cos(theta(a))) + (theta_k-theta(a))/(L_f*w_nom)*V(a)*V_s(a)*sin(theta(a));
    Aeq = eye(7,9);
    Beq = [w_nom; V_nom; omega_k; V_k; theta_k; P_k; Q_k ; 0; 0];
    
    H = zeros(9);
    H(1,1) = 2*lambda1(a);
    H(2,2) = 2*lambda2(a);
    H(6,6) = 2*lambda5(a)/Smax(a);
    H(7,7) = H(6,6)*lambda6(a)/lambda5(a);
    H(8,8) = 2*lambda3(a);
    H(9,9) = 2*lambda4(a);
    
    F = zeros(9,1);
    F(1,1) = -2*lambda1(a);
    F(2,1) = -2*lambda2(a);
    F(6,1) = -2*lambda5(a)*sum(aij(a,:)*P/Smax)*P(a)/Smax(a);
    F(7,1) = -2*lambda6(a)*sum(aij(a,:)*P/Smax)*P(a)/Smax(a);

    options = optimoptions('quadprog','Display','iter');

    [x, exitflag] = quadprog(H, F, Ai, Bi, Aeq, Beq, [], [], [], options);

    if exitflag > 0
        d_omega = x(8);
        d_V = x(9);
    else
        d_omega = 0;
        d_V = 0;
    end
    d_omega_old = d_omega;
    d_V_old = d_V;
    
end
